simulink model "simuss"  (R2024b)
settings: Solver=FixedStepAuto  StartTime=0.0  StopTime=0.03  FixedStep=0.00001  RelTol=1e-3
values from neighbouring files (symbols this model uses):
  A = [0, 1; -1/(L*Cap), -R/L]    [P4C.m]    (also in P4a.m = [0, 1;-1/(L*Cap),-R/L]; P4b.m = [0, 1;-1/(L*Cap),-R/L])
  B = [0; 1/L]    [P4C.m]    (also in P4a.m; P4b.m)
  C = [1/Cap, 1]    [P4C.m]    (also in P4a.m = [0 1]; P4b.m = [1/Cap 0])
  D = 0    [P4C.m]    (also in P4a.m; P4b.m)
settings Model: Creator=PROBOOK  LastModifiedBy=PROBOOK

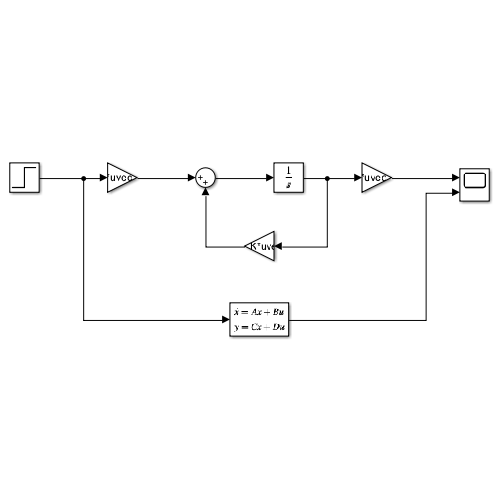
[thumbnail: Simulink's stored preview of the top-level diagram]
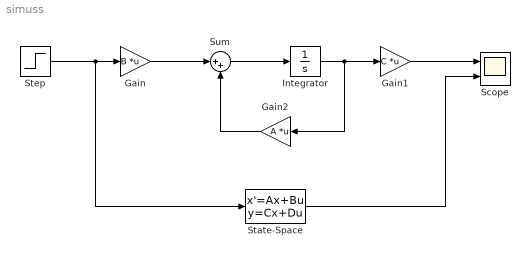
== system simuss ==
  Gain : Gain  Gain=B  Multiplication=Matrix(K*u) (u vector)
  Gain1 : Gain  Gain=C  Multiplication=Matrix(K*u) (u vector)
  Gain2 : Gain  Gain=A  Multiplication=Matrix(K*u) (u vector)
  Integrator : Integrator
  Scope : Scope  NumInputPorts=2
  State-Space : StateSpace  A=A  B=B  C=C  D=D  InitialCondition=0
  Step : Step  Time=0.01  SampleTime=0
  Sum : Sum  Inputs=|++
  wires:
  Step/1 -> State-Space/1, Gain/1
  Gain/1 -> Sum/1
  Sum/1 -> Integrator/1
  Integrator/1 -> Gain2/1, Gain1/1
  Gain2/1 -> Sum/2
  Gain1/1 -> Scope/1
  State-Space/1 -> Scope/2
